simulink model "untitled"  (R2019a)
settings: Solver=VariableStepAuto  StartTime=0.0  StopTime=10.0  RelTol=1e-3
libraries: aerolibanimutils x1
settings Model: Creator=m  LastModifiedBy=m

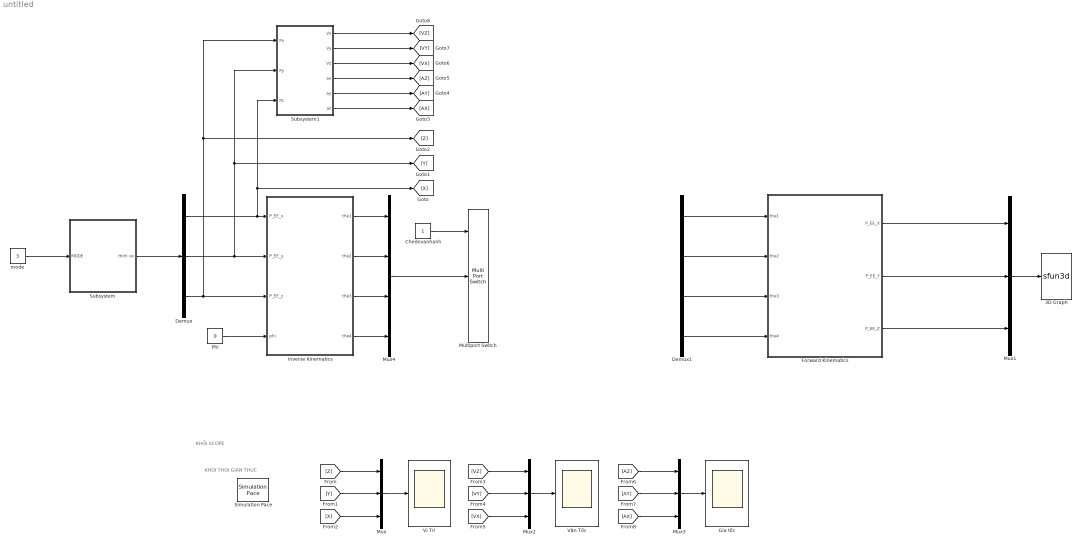
== system untitled ==
  note: KHOI THOi GIAN THUC
  note: KHỐI SCOPE
  3D Graph : S-Function  LoadFcn=if exist('sfun3d','file'), sfun3d([],[],[],'LoadBlock'); end  FunctionName=sfun3d  Parameters=ax,T,np,cp,gd,ls,mk,mx,hd,tb  SFunctionDeploymentMode=off  EnableBusSupport=off  mask(3D Graph){np=1, ax=[-500 1000 -500 1000 -500 1000], mx=1e4, T=0.01, cp=[3 2 1], gd=on, hd=off, tb=off, ls=:, mk=.}
      mask prompts: np "Number of moving points (lines)"; ax "Range: [xmin xmax  ymin ymax zmin zmax]"; mx "Max number of points in each line"; T "Sampling Time"; cp "Camera position (use [0 0 1] for 2D XY view)"; gd "Grid (on|off)"; hd "HeadMarkers (on|off)"; tb "Toolbar (on|off)"; ls "LineStyle"; mk "LineMarker"
      mask help:
      | This block plots the position of several points in the XYZ space. The input contains the coordinates of all the points (x1,y1,z1,x2,y2,z2,...).
      | The number of moving points (lines), the XYZ ranges, sampling time, camera position, and grid (among other things) can be set as mask parameters.
      settings: CopyFcn=if exist('sfun3d','file'), sfun3d([],[],[],'CopyBlock'); end  DeleteFcn=if exist('sfun3d','file'), sfun3d([],[],[],'DeleteBlock'); end  NameChangeFcn=if exist('sfun3d','file'), sfun3d([],[],[],'NameChange'); end
      mask Help:
      | This block plots the position of several points in the XYZ space. The input contains the coordinates of all the points (x1,y1,z1,x2,y2,z2,...).
      | The number of moving points (lines), the XYZ ranges, sampling time, camera position, and grid (among other things) can be set as mask parameters.
      mask TypeOptions ls: - | -- | : | -. | none
      mask TypeOptions mk: none | . | + | o | * | x | square | diamond | v | ^ | > | < | pentagram | hexagram
      mask Display: plot([.05 .95 .95 .05 .05],[.45 .45 .95 .95 .45], 0.5+cos(0:0.1:2*pi)*0.3,0.7+sin(0:0.1:2*pi)*0.2)
  Chedovanhanh : Constant
  Demux : Demux  Outputs=3
  Demux1 : Demux
  Forward Kinematics : MATLAB Function  TreatAsAtomicUnit=on
  Gia tốc : Scope
  Inverse Kinematics : MATLAB Function  TreatAsAtomicUnit=on
  Multiport Switch : MultiPortSwitch  Inputs=2
  Mux{,1..3} (4 alike) : Mux  Inputs=3
  Mux4 : Mux
  Phi : Constant  Value=0
  Simulation Pace : aerolibanimutils/Simulation Pace  SimulationPace=1  SleepMode=MATLAB Thread  OutputPaceError=off  SampleTime=0.01
  Subsystem : Subsystem
  Subsystem1 : Subsystem
  Vi Tri : Scope
  Vận Tốc : Scope
  mode : Constant  Value=3
  wires:
  Phi/1 -> Inverse Kinematics/4(phi)
  Subsystem1/3(Vz) -> [VX]
  Inverse Kinematics/4(the4) -> Mux4/4
  Demux/3 -> Inverse Kinematics/3(P_EE_z), Subsystem1/1(Px), [Z]
  Subsystem1/5(ay) -> [AY]
  Subsystem1/4(ax) -> [AZ]
  mode/1 -> Subsystem/1(MODE)
  Inverse Kinematics/3(the3) -> Mux4/3
  Subsystem1/1(Vx) -> [VZ]
  Demux/1 -> Subsystem1/3(Pz), [X], Inverse Kinematics/1(P_EE_x)
  Demux/2 -> Subsystem1/2(Py), [Y], Inverse Kinematics/2(P_EE_y)
  Subsystem1/2(Vy) -> [VY]
  Mux4/1 -> Multiport Switch/2
  Subsystem1/6(az) -> [AX]
  Inverse Kinematics/1(the1) -> Mux4/1
  Inverse Kinematics/2(the2) -> Mux4/2
  Chedovanhanh/1 -> Multiport Switch/1
  Subsystem/1(Hinh ve) -> Demux/1
  Mux2/1 -> Vận Tốc/1
  [AY] -> Mux3/2
  Mux/1 -> Vi Tri/1
  [Y] -> Mux/2
  [X] -> Mux/3
  [Z] -> Mux/1
  [AX] -> Mux3/3
  [VX] -> Mux2/3
  [AZ] -> Mux3/1
  [VY] -> Mux2/2
  Mux3/1 -> Gia tốc/1
  [VZ] -> Mux2/1
  Forward Kinematics/1(P_EE_X) -> Mux1/1
  Forward Kinematics/2(P_EE_Y) -> Mux1/2
  Forward Kinematics/3(P_EE_Z) -> Mux1/3
  Mux1/1 -> 3D Graph/1
  Demux1/1 -> Forward Kinematics/1(the1)
  Demux1/2 -> Forward Kinematics/2(the2)
  Demux1/3 -> Forward Kinematics/3(the3)
  Demux1/4 -> Forward Kinematics/4(the4)

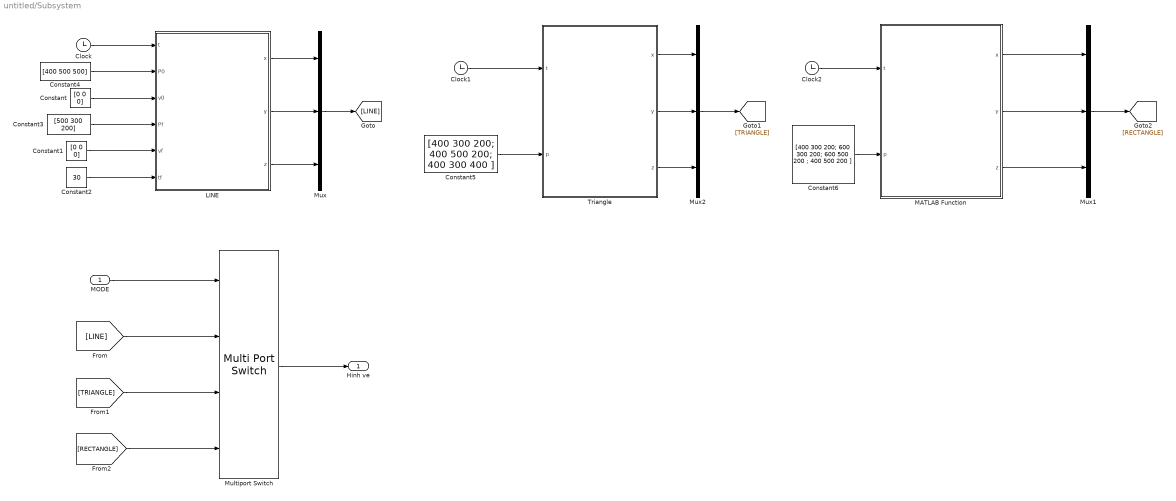
== system untitled/Subsystem ==
  MODE : Inport
  Clock : Clock
      settings: Decimation=30
  Clock1 : Clock
      settings: Decimation=30
  Clock2 : Clock
      settings: Decimation=40
  Constant : Constant  Value=[0 0 0]
  Constant1 : Constant  Value=[0 0 0]
  Constant2 : Constant  Value=30
  Constant3 : Constant  Value=[500 300 200]
  Constant4 : Constant  Value=[400 500 500]
  Constant5 : Constant  Value="[400 300 200; 400 500 200; 400 300 400  ]"
  Constant6 : Constant  Value=[400 300 200; 600 300 200; 600 500 200 ; 400 500 200 ]
  "LINE   " : MATLAB Function  TreatAsAtomicUnit=on
  MATLAB Function : MATLAB Function  TreatAsAtomicUnit=on
  Multiport Switch : MultiPortSwitch
  Mux : Mux  Inputs=3
  Mux1 : Mux  Inputs=3
  Mux2 : Mux  Inputs=3
  Triangle : MATLAB Function  TreatAsAtomicUnit=on
  Hinh ve : Outport
  wires:
  Clock1/1 -> Triangle/1(t)
  Constant4/1 -> "LINE   "/2(P0)
  Constant3/1 -> "LINE   "/4(Pf)
  Clock/1 -> "LINE   "/1(t)
  Constant2/1 -> "LINE   "/6(tf)
  Constant/1 -> "LINE   "/3(v0)
  Constant1/1 -> "LINE   "/5(vf)
  MODE/1 -> Multiport Switch/1
  "LINE   "/1(x) -> Mux/1
  "LINE   "/2(y) -> Mux/2
  "LINE   "/3(z) -> Mux/3
  Mux/1 -> [LINE]
  [LINE] -> Multiport Switch/2
  [TRIANGLE] -> Multiport Switch/3
  [RECTANGLE] -> Multiport Switch/4
  Triangle/1(x) -> Mux2/1
  Triangle/2(y) -> Mux2/2
  Mux2/1 -> [TRIANGLE]
  Triangle/3(z) -> Mux2/3
  Constant5/1 -> Triangle/2(p)
  Mux1/1 -> [RECTANGLE]
  MATLAB Function/1(x) -> Mux1/1
  MATLAB Function/2(y) -> Mux1/2
  MATLAB Function/3(z) -> Mux1/3
  Clock2/1 -> MATLAB Function/1(t)
  Constant6/1 -> MATLAB Function/2(p)
  Multiport Switch/1 -> Hinh ve/1

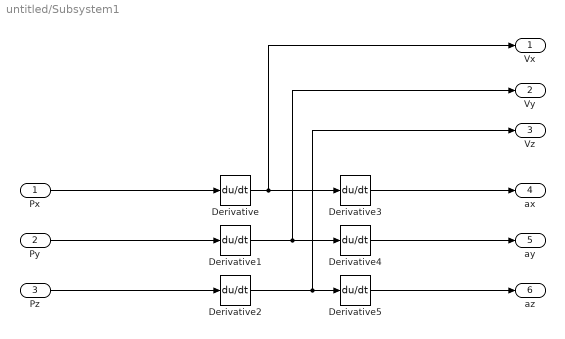
== system untitled/Subsystem1 ==
  Px : Inport
  Py : Inport  Port=2
  Pz : Inport  Port=3
  Derivative{,1..5} (6 alike) : Derivative
  Vx : Outport
  Vy : Outport  Port=2
  Vz : Outport  Port=3
  ax : Outport  Port=4
  ay : Outport  Port=5
  az : Outport  Port=6
  wires:
  Derivative4/1 -> ay/1
  Px/1 -> Derivative/1
  Py/1 -> Derivative1/1
  Pz/1 -> Derivative2/1
  Derivative5/1 -> az/1
  Derivative2/1 -> Vz/1, Derivative5/1
  Derivative/1 -> Vx/1, Derivative3/1
  Derivative1/1 -> Vy/1, Derivative4/1
  Derivative3/1 -> ax/1

== matlab function untitled/Inverse Kinematics ==
  data: P_EE_x input; P_EE_y input; P_EE_z input; the1 output; phi input; the2 output; the3 output; the4 output
function [the1,the2,the3,the4]=IK_4DOF(P_EE_x,P_EE_y,P_EE_z,phi)
l1=150; l2=350; l3=363.5; l4=210;
d1=140;
 % tim the1
the1=atan2d(P_EE_y,P_EE_x);
Px=P_EE_x-l4*cosd(the1)*cosd(phi);
Py=P_EE_y-l4*sind(the1)*cosd(phi);
Pz=P_EE_z+l4*sind(phi);

 %tim theta3 >0
 nx=Px*cosd(the1)+Py*sind(the1)-l1;
 ny=Pz-d1;
 c3=(nx*nx+ny*ny-l3*l3-l2*l2)/(2*l2*l3);
 s3=sqrt(1-c3^2);
 the3=atan2d(s3,c3);
 %tim theta2 >0;
 the2=atan2d(-((ny*(l3*cosd(the3)+l2)+l3*sind(the3)*nx)),-((-nx*(l3*cosd(the3)+l2)+l3*sind(the3)*ny)));
 %tim theta4 
 the4=phi-the2-the3;

== matlab function untitled/Forward Kinematics ==
  data: the1 input; P_EE_X output; the2 input; the3 input; the4 input; P_EE_Y output; P_EE_Z output
function [P_EE_X,P_EE_Y,P_EE_Z]=FK_4DOF(the1,the2,the3,the4)
l1=150; l2=350; l3=363.5; l4=210;
d1=140;
P_EE_X=cosd(the1)*(l1+l3*cosd(the2+the3)+l2*cosd(the2)+l4*cosd(the2+the3+the4));
P_EE_Y=sind(the1)*(l1+l3*cosd(the2+the3)+l2*cosd(the2)+l4*cosd(the2+the3+the4));
P_EE_Z=d1-l3*sind(the2+the3)-l2*sind(the2)-l4*sind(the2+the3+the4);
end

== matlab function untitled/Subsystem/LINE    ==
  data: x output; t input; y output; P0 input; v0 input; Pf input; vf input; tf input; z output
function [x,y,z] = LINE(t,P0,v0,Pf,vf,tf)
a10=P0(1);
a20=P0(2);
a30=P0(3);
a11=v0(1);
a21=v0(2);
a31=v0(3);
a12=3/tf^2*(Pf(1)-P0(1))-2/tf*v0(1)-1/tf*vf(1);
a22=3/tf^2*(Pf(2)-P0(2))-2/tf*v0(2)-1/tf*vf(2);
a32=3/tf^2*(Pf(3)-P0(3))-2/tf*v0(3)-1/tf*vf(3);
a13=-2/tf^3*(Pf(1)-P0(1))+1/tf^2*(vf(1)+v0(1));
a23=-2/tf^3*(Pf(2)-P0(2))+1/tf^2*(vf(2)+v0(2));
a33=-2/tf^3*(Pf(3)-P0(3))+1/tf^2*(vf(3)+v0(3));
if t<30
    x=a10+a11*t+a12*t^2+a13*t^3;
    y=a20+a21*t+a22*t^2+a23*t^3;
    z=a30+a31*t+a32*t^2+a33*t^3; 
else
    t=30;
    x=a10+a11*t+a12*t^2+a13*t^3;
    y=a20+a21*t+a22*t^2+a23*t^3;
    z=a30+a31*t+a32*t^2+a33*t^3; 
end

== matlab function untitled/Subsystem/Triangle ==
  data: x output; t input; y output; p input; z output
function [x,y,z] = Triangle(t,p)
t0=0;
tf=10;
t1=t;
v0=0;
vf=0;
%Phương trình quĩ đạo bậc 3: P(t) = a0 + a1*t+ a2*t^2 + a3*t^3
A=[ 1 t0 t0^2 t0^3;
    0  1  2*t0 3*t0^2; 
    1 tf tf^2 tf^3;
    0 1  2*tf 3*tf^2;];
if t<=10
%%
C=[ p(1,1); v0; p(2,1); vf];
Bx=A\C;
x = Bx(1,1) + Bx(2,1)*t1 +Bx(3,1)*t1^2 + Bx(4,1)*t1^3;
C=[p(1,2); v0; p(2,2); vf];
By=A\C;
y = By(1,1) + By(2,1)*t1 +By(3,1)*t1^2 + By(4,1)*t1^3;
C=[p(1,3); v0; p(2,3); vf];
Bz=A\C;
z = Bz(1,1) + Bz(2,1)*t1 +Bz(3,1)*t1^2 + Bz(4,1)*t1^3;
elseif (t>10)&&(t<=20)
t1=t1-10;
C=[ p(2,1); v0; p(3,1); vf];
Bx=A\C;
x = Bx(1,1) + Bx(2,1)*t1 +Bx(3,1)*t1^2 + Bx(4,1)*t1^3;
C=[ p(2,2); v0; p(3,2); vf];
By=A\C;
y = By(1,1) + By(2,1)*t1 +By(3,1)*t1^2 + By(4,1)*t1^3;

C=[ p(2,3); v0; p(3,3); vf];
Bz=A\C;
z = Bz(1,1) + Bz(2,1)*t1 +Bz(3,1)*t1^2 + Bz(4,1)*t1^3;
elseif t<30
t1=t1-20;
C=[p(3,1); v0; p(1,1); vf];
Bx=A\C;
x = Bx(1,1) + Bx(2,1)*t1 +Bx(3,1)*t1^2 + Bx(4,1)*t1^3;
C=[ p(3,2); v0; p(1,2); vf];
By=A\C;
y = By(1,1) + By(2,1)*t1 +By(3,1)*t1^2 + By(4,1)*t1^3;

C=[ p(3,3); v0; p(1,3); vf];
Bz=A\C;
z = Bz(1,1) + Bz(2,1)*t1 +Bz(3,1)*t1^2 + Bz(4,1)*t1^3;
else
t1=30;
t1=t1-20;
C=[p(3,1); v0; p(1,1); vf];
Bx=A\C;
x = Bx(1,1) + Bx(2,1)*t1 +Bx(3,1)*t1^2 + Bx(4,1)*t1^3;
C=[ p(3,2); v0; p(1,2); vf];
By=A\C;
y = By(1,1) + By(2,1)*t1 +By(3,1)*t1^2 + By(4,1)*t1^3;
C=[ p(3,3); v0; p(1,3); vf];
Bz=A\C;
z = Bz(1,1) + Bz(2,1)*t1 +Bz(3,1)*t1^2 + Bz(4,1)*t1^3;
end

== matlab function untitled/Subsystem/MATLAB Function ==
  data: x output; t input; y output; p input; z output
function [x,y,z] = Rectangle(t,p)
t0=0;
tf=10;
t1=t;
v0=0;
vf=0;
%Phương trình quĩ đạo bậc 3: P(t) = a0 + a1*t+ a2*t^2 + a3*t^3
A=[ 1 t0 t0^2 t0^3;
    0  1  2*t0 3*t0^2; 
    1 tf tf^2 tf^3;
    0 1  2*tf 3*tf^2;];
if t<=10
%%
C=[ p(1,1); v0; p(2,1); vf];
Bx=A\C;
x = Bx(1,1) + Bx(2,1)*t1 +Bx(3,1)*t1^2 + Bx(4,1)*t1^3;
C=[p(1,2); v0; p(2,2); vf];
By=A\C;
y = By(1,1) + By(2,1)*t1 +By(3,1)*t1^2 + By(4,1)*t1^3;
C=[p(1,3); v0; p(2,3); vf];
Bz=A\C;
z = Bz(1,1) + Bz(2,1)*t1 +Bz(3,1)*t1^2 + Bz(4,1)*t1^3;
elseif (t>10)&&(t<=20)
t1=t1-10;
C=[ p(2,1); v0; p(3,1); vf];
Bx=A\C;
x = Bx(1,1) + Bx(2,1)*t1 +Bx(3,1)*t1^2 + Bx(4,1)*t1^3;
C=[ p(2,2); v0; p(3,2); vf];
By=A\C;
y = By(1,1) + By(2,1)*t1 +By(3,1)*t1^2 + By(4,1)*t1^3;

C=[ p(2,3); v0; p(3,3); vf];
Bz=A\C;
z = Bz(1,1) + Bz(2,1)*t1 +Bz(3,1)*t1^2 + Bz(4,1)*t1^3;
elseif (t>20)&&(t<=30) 
t1=t1-20;
C=[p(3,1); v0; p(4,1); vf];
Bx=A\C;
x = Bx(1,1) + Bx(2,1)*t1 +Bx(3,1)*t1^2 + Bx(4,1)*t1^3;
C=[ p(3,2); v0; p(4,2); vf];
By=A\C;
y = By(1,1) + By(2,1)*t1 +By(3,1)*t1^2 + By(4,1)*t1^3;

C=[ p(3,3); v0; p(4,3); vf];
Bz=A\C;
z = Bz(1,1) + Bz(2,1)*t1 +Bz(3,1)*t1^2 + Bz(4,1)*t1^3;

elseif t1<=40
t1=t1-30;
C=[p(4,1); v0; p(1,1); vf];
Bx=A\C;
x = Bx(1,1) + Bx(2,1)*t1 +Bx(3,1)*t1^2 + Bx(4,1)*t1^3;
C=[ p(4,2); v0; p(1,2); vf];
By=A\C;
y = By(1,1) + By(2,1)*t1 +By(3,1)*t1^2 + By(4,1)*t1^3;

C=[ p(4,3); v0; p(1,3); vf];
Bz=A\C;
z = Bz(1,1) + Bz(2,1)*t1 +Bz(3,1)*t1^2 + Bz(4,1)*t1^3;
else
t1=40;
t1=t1-30;
C=[p(4,1); v0; p(1,1); vf];
Bx=A\C;
x = Bx(1,1) + Bx(2,1)*t1 +Bx(3,1)*t1^2 + Bx(4,1)*t1^3;
C=[ p(4,2); v0; p(1,2); vf];
By=A\C;
y = By(1,1) + By(2,1)*t1 +By(3,1)*t1^2 + By(4,1)*t1^3;

C=[ p(4,3); v0; p(1,3); vf];
Bz=A\C;
z = Bz(1,1) + Bz(2,1)*t1 +Bz(3,1)*t1^2 + Bz(4,1)*t1^3;
end
